simulink model "test"  (R2017a)
settings: Solver=VariableStepAuto  StartTime=0.0  StopTime=10.0  RelTol=1e-3
model workspace: external: MAT-File C:\Users\calvinv\Google Drive\code\Matlab\QuadSim\Simulink\parameters\param.mat (data not in the file)
libraries: simulink x2
settings Model: Creator=calvin  LastModifiedBy=calvin

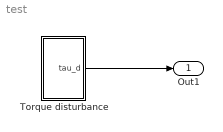
== system test ==
  Torque disturbance : Subsystem  mask{d=0}
      mask prompts: d "Disturbance magnitude"
  Out1 : Outport
  wires:
  Torque disturbance/1(tau_d) -> Out1/1

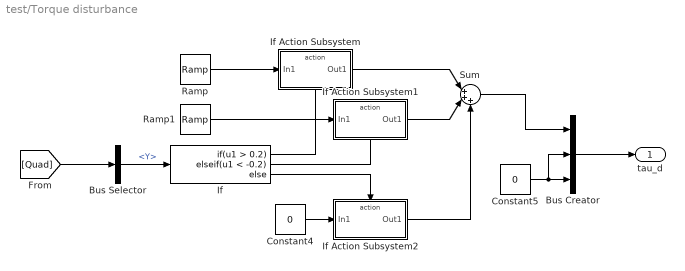
== system test/Torque disturbance ==
  Bus Creator : BusCreator  Inputs=3
  Bus Selector : BusSelector  OutputSignals=Y
  Constant4 : Constant  Value=0
  Constant5 : Constant  Value=0
  If : If  IfExpression=u1 > 0.2  ElseIfExpressions=u1 < -0.2
  If Action Subsystem : Subsystem  TreatAsAtomicUnit=on
  If Action Subsystem1 : Subsystem  TreatAsAtomicUnit=on
  If Action Subsystem2 : Subsystem  TreatAsAtomicUnit=on
  Ramp : simulink/Sources/Ramp  slope=-d  start=0  X0=0
  Ramp1 : simulink/Sources/Ramp  slope=d  start=0  X0=0
  Sum : Sum  Inputs=|+++
  tau_d : Outport
  wires:
  [Quad] -> Bus Selector/1
  Bus Selector/1 -> If/1  "<Y>"
  Ramp1/1 -> If Action Subsystem1/1(In1)
  Ramp/1 -> If Action Subsystem/1(In1)
  Bus Creator/1 -> tau_d/1
  If/3 -> If Action Subsystem2/Action
  If Action Subsystem2/1(Out1) -> Sum/3
  If/1 -> If Action Subsystem/Action
  If Action Subsystem1/1(Out1) -> Sum/2
  If/2 -> If Action Subsystem1/Action
  Constant5/1 -> Bus Creator/2, Bus Creator/3
  If Action Subsystem/1(Out1) -> Sum/1
  Sum/1 -> Bus Creator/1
  Constant4/1 -> If Action Subsystem2/1(In1)

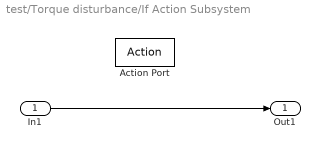
== system test/Torque disturbance/If Action Subsystem ==
  In1 : Inport
  Action Port : ActionPort  ActionType=then
  Out1 : Outport
  wires:
  In1/1 -> Out1/1

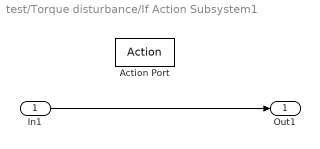
== system test/Torque disturbance/If Action Subsystem1 ==
  In1 : Inport
  Action Port : ActionPort  ActionType=elseif
  Out1 : Outport
  wires:
  In1/1 -> Out1/1

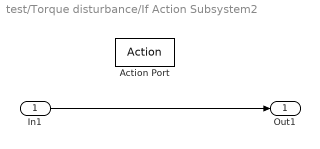
== system test/Torque disturbance/If Action Subsystem2 ==
  In1 : Inport
  Action Port : ActionPort  ActionType=else
  Out1 : Outport
  wires:
  In1/1 -> Out1/1
